simulink model "sim_kalman_dcorr_internal"  (Simulink 8.5)
settings: Solver=ode23s  StartTime=0.0  StopTime=2*max(time)  FixedStep=0.0001  RelTol=1e-3
values from neighbouring files (symbols this model uses):
  CTRL = ctrl_d(i)    [step3_analyse_export.m]    (also in step4_simulation.m = ctrl_d(5))
  Pd00 = eye(CTRL.n + CTRL.m, CTRL.n + CTRL.m)*1e3    [step4_simulation.m]
  PLANT = model.chip    [step2_design_controller.m]    (also in step3_analyse_export.m = model.combo; step4_simulation.m = model.combo)
  RESET_TIME = REFERENCE_STEP_DURATION*(1 + length(CTRL.output))    [step4_simulation.m]
  Rv = eye(CTRL.p,CTRL.p)*(DOUBT_SENSOR^2/12)    [step4_simulation.m]
  WdRwWd = CTRL.Wd * Rw * CTRL.Wd'    [step4_simulation.m]
libraries: simulink x5
settings Model: Creator=yh3wong  LastModifiedBy=yh3wong  CovSFcnEnable=off
settings DataIOCC: SignalLoggingSaveFormat=Dataset
settings OptimizationCC: ExpressionDepthLimit=128
settings DebuggingCC: UnderspecifiedInitializationDetection=Simplified  MergeDetectMultiDrivingBlocksExec=error  SolverPrmCheckMsg=warning  FcnCallInpInsideContextMsg=EnableAllAsError  StateNameClashWarn=none
settings GRTTargetCC: CombineOutputUpdateFcns=on  GRTInterface=off

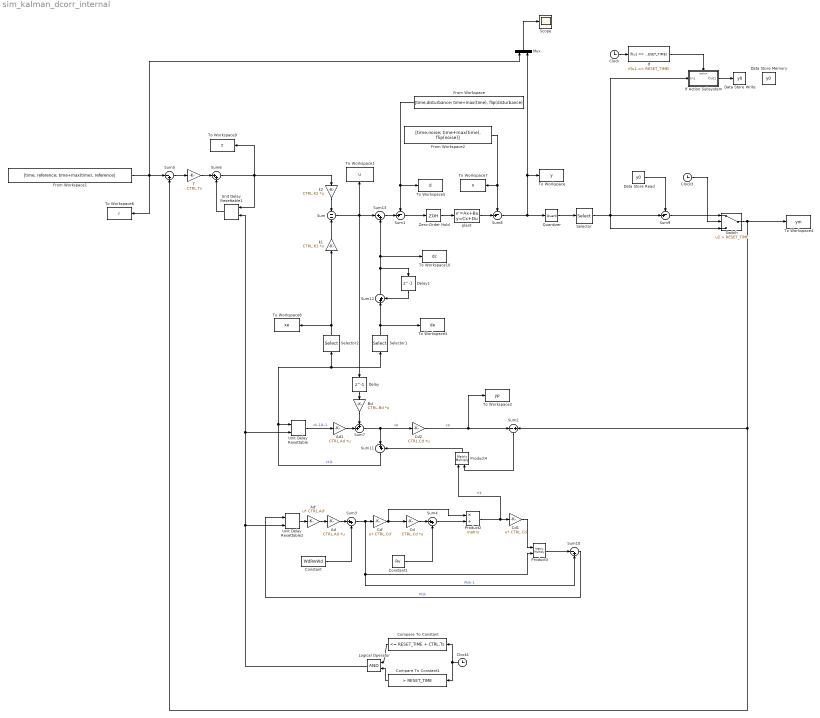
== system sim_kalman_dcorr_internal ==
  Ad : Gain  Gain=CTRL.Ad  Multiplication=Matrix(K*u)  SampleTime=CTRL.Ts
  Ad' : Gain  Gain=CTRL.Ad'  Multiplication=Matrix(u*K)  SampleTime=CTRL.Ts
  Ad1 : Gain  Gain=CTRL.Ad  Multiplication=Matrix(K*u)  SampleTime=CTRL.Ts
  Bd : Gain  Gain=CTRL.Bd  Multiplication=Matrix(K*u)  SampleTime=CTRL.Ts
  Cd : Gain  Gain=CTRL.Cd  Multiplication=Matrix(K*u)  SampleTime=CTRL.Ts
  Cd' : Gain  Gain=CTRL.Cd'  Multiplication=Matrix(u*K)  SampleTime=CTRL.Ts
  Cd1 : Gain  Gain=CTRL.Cd  Multiplication=Matrix(u*K)  SampleTime=CTRL.Ts
  Cd2 : Gain  Gain=CTRL.Cd  Multiplication=Matrix(K*u)  SampleTime=CTRL.Ts
  Clock : Clock
  Clock1 : Clock
  Clock3 : Clock
  Compare To Constant : simulink/Logic and Bit Operations/Compare To Constant  relop=<=  const=RESET_TIME + CTRL.Ts  OutDataTypeStr=boolean
  Compare To Constant1 : simulink/Logic and Bit Operations/Compare To Constant  relop=>  const=RESET_TIME  OutDataTypeStr=boolean
  Constant : Constant  Value=WdRwWd  VectorParams1D=off
  Constant1 : Constant  Value=Rv  VectorParams1D=off
  Data Store Memory : DataStoreMemory  DataStoreName=y0  ReadBeforeWriteMsg=error  WriteAfterWriteMsg=error  WriteAfterReadMsg=error  InitialValue=zeros(size(CTRL.output))
  Data Store Read : DataStoreRead  DataStoreName=y0  SampleTime=CTRL.Ts
  Data Store Write : DataStoreWrite  DataStoreName=y0
  Delay : Delay  DelayLength=1  InitialCondition=0
  Delay1 : Delay  DelayLength=1  InitialCondition=0
  From Workspace : FromWorkspace  VariableName=[time,disturbance; time+max(time), flip(disturbance)]  SampleTime=CTRL.Ts  Interpolate=off  OutputAfterFinalValue=Holding final value
  From Workspace1 : FromWorkspace  VariableName=[time, reference; time+max(time), reference]  SampleTime=CTRL.Ts  Interpolate=off  OutputAfterFinalValue=Holding final value
  From Workspace2 : FromWorkspace  VariableName=[time,noise; time+max(time), flip(noise)]  SampleTime=CTRL.Ts  OutputAfterFinalValue=Holding final value
  If : If  IfExpression=u1 == RESET_TIME  ShowElse=off
  If Action Subsystem : Subsystem  TreatAsAtomicUnit=on
  Logical Operator : Logic  AllPortsSameDT=off  OutDataTypeStr=boolean
  Mux : Mux  Inputs=2
  Product2 : Product  Inputs=*/  Multiplication=Matrix(*)  SampleTime=CTRL.Ts
  Product3 : Product  Inputs=**  Multiplication=Matrix(*)  SampleTime=CTRL.Ts
  Product4 : Product  Inputs=**  Multiplication=Matrix(*)  SampleTime=CTRL.Ts
  Quantizer : Quantizer  QuantizationInterval=DOUBT_SENSOR
  Scope : Scope
      settings: YMin=-150  YMax=200
  Selector : Selector  InputPortWidth=length(PLANT.output)  Indices=CTRL.channel_idx
  Selector1 : Selector  InputPortWidth=length(CTRL.state_d)  Indices=disturbance_idx
  Selector2 : Selector  InputPortWidth=length(CTRL.state_d)  Indices=state_idx
  Sum : Sum  Inputs=-|-  SampleTime=CTRL.Ts
  Sum1 : Sum  Inputs=-+|  SampleTime=CTRL.Ts
  Sum10 : Sum  Inputs=|-+  SampleTime=CTRL.Ts
  Sum{3..4,6,11..13} (6 alike) : Sum  Inputs=|++  SampleTime=CTRL.Ts
  Sum2 : Sum  Inputs=-|+  SampleTime=CTRL.Ts
  Sum5 : Sum  Inputs=|-+  SampleTime=CTRL.Ts
  Sum7 : Sum  Inputs=++|  SampleTime=CTRL.Ts
  Sum8 : Sum  Inputs=-+|
  Sum9 : Sum  Inputs=-+|  SampleTime=CTRL.Ts
  Switch : Switch  Criteria=u2 > Threshold  Threshold=RESET_TIME  SampleTime=CTRL.Ts
  T : Gain  Gain=CTRL.Ts  SampleTime=CTRL.Ts
  To Workspace : ToWorkspace  VariableName=y  SaveFormat=Structure With Time  SampleTime=-1
  To Workspace1 : ToWorkspace  VariableName=u  SaveFormat=Structure With Time  SampleTime=CTRL.Ts
  To Workspace10 : ToWorkspace  VariableName=dc  SaveFormat=Structure With Time  SampleTime=CTRL.Ts
  To Workspace2 : ToWorkspace  VariableName=yp  SaveFormat=Structure With Time  SampleTime=CTRL.Ts
  To Workspace3 : ToWorkspace  VariableName=de  SaveFormat=Structure With Time  SampleTime=CTRL.Ts
  To Workspace4 : ToWorkspace  VariableName=ym  SaveFormat=Structure With Time  SampleTime=-1
  To Workspace5 : ToWorkspace  VariableName=d  SaveFormat=Structure With Time  SampleTime=CTRL.Ts
  To Workspace6 : ToWorkspace  VariableName=r  SaveFormat=Structure With Time  SampleTime=CTRL.Ts
  To Workspace7 : ToWorkspace  VariableName=n  SaveFormat=Structure With Time  SampleTime=CTRL.Ts
  To Workspace8 : ToWorkspace  VariableName=xe  SaveFormat=Structure With Time  SampleTime=CTRL.Ts
  To Workspace9 : ToWorkspace  VariableName=z  SaveFormat=Structure With Time  SampleTime=CTRL.Ts
  Unit Delay Resettable : simulink/Additional Math & Discrete/Additional Discrete/Unit Delay Resettable  vinit=zeros(size(CTRL.state_d))  tsamp=CTRL.Ts
  Unit Delay Resettable1 : simulink/Additional Math & Discrete/Additional Discrete/Unit Delay Resettable  vinit=zeros(size(CTRL.output))  tsamp=CTRL.Ts
  Unit Delay Resettable2 : simulink/Additional Math & Discrete/Additional Discrete/Unit Delay Resettable  vinit=Pd00  tsamp=CTRL.Ts
  Zero-Order Hold : ZeroOrderHold  SampleTime=CTRL.Ts
  "k1 " : Gain  Gain=CTRL.K1  Multiplication=Matrix(K*u)  SampleTime=CTRL.Ts
  k2 : Gain  Gain=CTRL.K2  Multiplication=Matrix(K*u)  SampleTime=CTRL.Ts
  plant : StateSpace  A=PLANT.Ac  B=PLANT.Bc  C=PLANT.Cc  D=PLANT.Dc  X0=0
  wires:
  k2/1 -> Sum/1
  "k1 "/1 -> Sum/2
  Zero-Order Hold/1 -> plant/1
  From Workspace/1 -> Sum1/1, To Workspace5/1
  Sum1/1 -> Zero-Order Hold/1
  Sum5/1 -> T/1
  plant/1 -> Sum8/2
  From Workspace1/1 -> To Workspace6/1, Sum5/1, Mux/1
  Mux/1 -> Scope/1
  Sum8/1 -> Quantizer/1, To Workspace/1, Mux/2
  If/1 -> If Action Subsystem/Action
  If Action Subsystem/1(Out1) -> Data Store Write/1
  Switch/1 -> To Workspace4/1, Sum2/2, Sum5/2
  Sum9/1 -> Switch/1
  Data Store Read/1 -> Sum9/1
  Clock1/1 -> Compare To Constant/1, Compare To Constant1/1
  Compare To Constant/1 -> Logical Operator/1
  Compare To Constant1/1 -> Logical Operator/2
  Clock/1 -> If/1
  Clock3/1 -> Switch/2
  Selector/1 -> If Action Subsystem/1(In1), Switch/3, Sum9/2
  From Workspace2/1 -> To Workspace7/1, Sum8/1
  Unit Delay Resettable2/1 -> Ad'/1
  Ad'/1 -> Ad/1
  Sum10/1 -> Unit Delay Resettable2/1  "Pk|k"
  Sum3/1 -> Product3/2, Sum10/2, Cd'/1  "Pk|k-1"
  Cd'/1 -> Cd/1, Product2/1
  Sum4/1 -> Product2/2
  Product2/1 -> Cd1/1, Product4/1  "Kk"
  Cd2/1 -> Sum2/1, To Workspace2/1  "yp"
  Unit Delay Resettable/1 -> Ad1/1  "xk-1|k-1"
  Ad1/1 -> Sum7/2
  Bd/1 -> Sum7/1
  Sum7/1 -> Cd2/1, Sum11/1  "xp"
  Sum11/1 -> Unit Delay Resettable/1, Selector1/1, Selector2/1  "xk|k"
  Delay/1 -> Bd/1
  Quantizer/1 -> Selector/1
  Selector2/1 -> To Workspace8/1, "k1 "/1
  Sum/1 -> Sum13/1, Delay/1, To Workspace1/1
  Sum13/1 -> Sum1/2
  Cd1/1 -> Product3/1
  Product3/1 -> Sum10/1
  Cd/1 -> Sum4/1
  Constant1/1 -> Sum4/2
  Ad/1 -> Sum3/1
  Constant/1 -> Sum3/2
  Sum2/1 -> Product4/2
  Product4/1 -> Sum11/2
  T/1 -> Sum6/1
  Unit Delay Resettable1/1 -> Sum6/2
  Sum6/1 -> k2/1, To Workspace9/1, Unit Delay Resettable1/1
  Logical Operator/1 -> Unit Delay Resettable2/2, Unit Delay Resettable/2, Unit Delay Resettable1/2
  Delay1/1 -> Sum12/2
  Sum12/1 -> To Workspace10/1, Sum13/2, Delay1/1
  Selector1/1 -> Sum12/1, To Workspace3/1

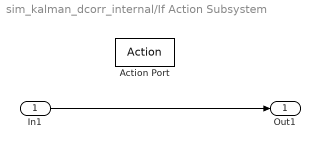
== system sim_kalman_dcorr_internal/If Action Subsystem ==
  In1 : Inport
  Action Port : ActionPort  ActionType=then
  Out1 : Outport
  wires:
  In1/1 -> Out1/1
